simulink model "Ej2"  (R2025b)
settings: Solver=VariableStepAuto  StartTime=0.0  StopTime=10.0  RelTol=1e-3
libraries: commrandsrc3 x1, dspfdesign x1
settings Model: Creator=Henry  LastModifiedBy=Henry

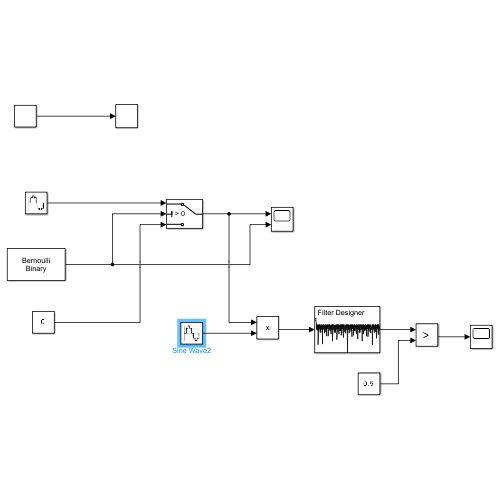
[thumbnail: Simulink's stored preview of the top-level diagram]
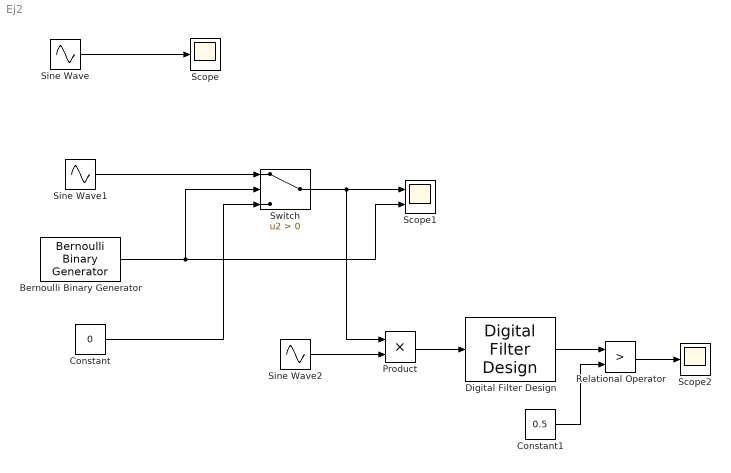
== system Ej2 ==
  Bernoulli Binary Generator : commrandsrc3/Bernoulli Binary Generator  ProbabilityOfZero=0.5  SeedSource=Auto  Seed=0  SampleTime=1  SamplesPerFrame=1  OutputDataType=double  SimulateUsing=Interpreted execution
  Constant : Constant  Value=0
  Constant1 : Constant  Value=0.5
  Digital Filter Design : dspfdesign/Digital Filter Design  mwdsp_browser_bugfix_var=off
  Product : Product
  Relational Operator : RelationalOperator  Operator=>  OutDataTypeStr=boolean  RndMeth=Simplest  InputSameDT=off
  Scope : Scope
      settings: ActiveDisplayYMinimum=-1.2456318853205086  ActiveDisplayYMaximum=1.2490408795261734
  Scope1 : Scope  NumInputPorts=2
      settings: ActiveDisplayYMinimum=-1.2475334105405018  ActiveDisplayYMaximum=1.2475334105405003
  Scope2 : Scope
      settings: ActiveDisplayYMinimum=-0.12499999999999997  ActiveDisplayYMaximum=1.125  DataLoggingVariableName=ScopeData2
  Sine Wave : Sin  SampleTime=0
  Sine Wave1 : Sin  Frequency=2*pi*100  SampleTime=0.0001
  Sine Wave2 : Sin  Frequency=2*pi*100  SampleTime=0.0001
  Switch : Switch  Criteria=u2 > Threshold  SaturateOnIntegerOverflow=off  InputSameDT=off
  wires:
  Sine Wave/1 -> Scope/1
  Sine Wave1/1 -> Switch/1
  Bernoulli Binary Generator/1 -> Scope1/2, Switch/2
  Constant/1 -> Switch/3
  Switch/1 -> Product/1, Scope1/1
  Sine Wave2/1 -> Product/2
  Product/1 -> Digital Filter Design/1
  Digital Filter Design/1 -> Relational Operator/1
  Constant1/1 -> Relational Operator/2
  Relational Operator/1 -> Scope2/1
